simulink model "Linear_Control_Lab_Lab2_DC_Motor_Model"  (R2018b)
settings: Solver=VariableStepAuto  StartTime=0.0  StopTime=10.0  RelTol=1e-3
values from neighbouring files (symbols this model uses):
  B = 3.5077e-06    [Linear_Control_Lab_Lab2_DC_Motor.mat]
  J = 3.2284e-05    [Linear_Control_Lab_Lab2_DC_Motor.mat]
  K = 0.0274    [Linear_Control_Lab_Lab2_DC_Motor.mat]
  L = 2.75e-06    [Linear_Control_Lab_Lab2_DC_Motor.mat]
  R = 4    [Linear_Control_Lab_Lab2_DC_Motor.mat]
settings Model: Creator=HP  LastModifiedBy=HP

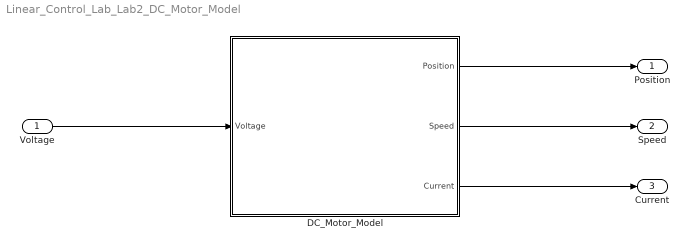
== system Linear_Control_Lab_Lab2_DC_Motor_Model ==
  Voltage : Inport
  DC_Motor_Model : Subsystem
  Position : Outport
  Speed : Outport  Port=2
  Current : Outport  Port=3
  wires:
  DC_Motor_Model/2(Speed) -> Speed/1
  DC_Motor_Model/1(Position) -> Position/1
  Voltage/1 -> DC_Motor_Model/1(Voltage)
  DC_Motor_Model/3(Current) -> Current/1

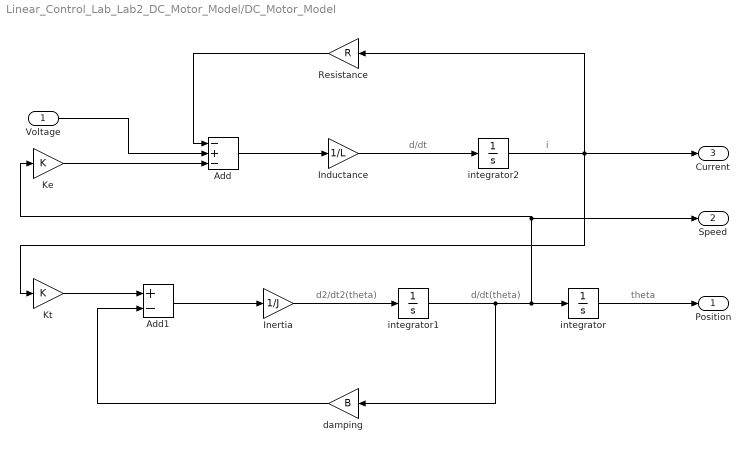
== system Linear_Control_Lab_Lab2_DC_Motor_Model/DC_Motor_Model ==
  note: i
  note: d2/dt2(theta)
  note: d/dt
  note: theta
  note: d/dt(theta)
  Voltage : Inport
  "Add " : Sum  Inputs=-+-
  "Add1 " : Sum  Inputs=+-
  Inductance : Gain  Gain=1/L
  Inertia : Gain  Gain=1/J
  Ke : Gain  Gain=K
  Kt : Gain  Gain=K
  Resistance : Gain  Gain=R
  damping : Gain  Gain=B
  integrator : Integrator
  "integrator1 " : Integrator
  integrator2 : Integrator
  Position : Outport
  Speed : Outport  Port=2
  Current : Outport  Port=3
  wires:
  Inductance/1 -> integrator2/1
  Inertia/1 -> "integrator1 "/1
  "Add "/1 -> Inductance/1
  integrator2/1 -> Current/1, Resistance/1, Kt/1
  Kt/1 -> "Add1 "/1
  "integrator1 "/1 -> damping/1, Speed/1, Ke/1, integrator/1
  integrator/1 -> Position/1
  damping/1 -> "Add1 "/2
  "Add1 "/1 -> Inertia/1
  Voltage/1 -> "Add "/2
  Ke/1 -> "Add "/3
  Resistance/1 -> "Add "/1
